simulink library "mylib"  (Simulink 9.2)
settings: Solver=VariableStepAuto  StartTime=0.0  StopTime=10.0  RelTol=1e-3
values from neighbouring files (symbols this model uses):
  FLINT32_MAX = flintmax('single')    [lib_consts.m]
undefined symbols (not defined in the file or in its folder): BAR_2_Pa, CC_2_M3, CCpREV_2_M3pRAD, DEG_2_RAD, DiscIntNeverNeededParam, G_2_MPS2, KNOTS_2_KPH, KPH_2_KNOTS, KPH_2_MPS, kXX_2_XX, M3_2_CC, M3pRAD_2_CCpREV, MPS2_2_G, MPS_2_KPH, Pa_2_BAR, RAD_2_DEG, RADpS_2_RPM, RPM_2_RADpS, XX_2_kXX
libraries: $bdroot x12, simulink x4, Ricardo_SW_dev_lib x1
(part 1 of 2)
settings Model: Creator=Gavin  LastModifiedBy=Gavin

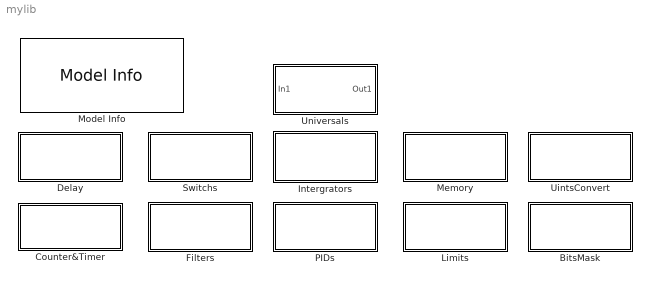
== system mylib ==
  BitsMask : Subsystem
      mask Display:
      | name = gcb;
      | str_id = strfind(gcb,'/');
      | name_mask = name(str_id+1:end);
      | disp([name_mask,'\nBlocks']);
      | color('black')
  Counter&Timer : Subsystem
      mask Display:
      | name = gcb;
      | str_id = strfind(gcb,'/');
      | name_mask = name(str_id+1:end);
      | disp([name_mask,'\nBlocks']);
      | color('black')
  Delay : Subsystem
      mask Display:
      | name = gcb;
      | str_id = strfind(gcb,'/');
      | name_mask = name(str_id+1:end);
      | disp([name_mask,'\nBlocks']);
      | color('black')
  Filters : Subsystem
      mask Display:
      | name = gcb;
      | str_id = strfind(gcb,'/');
      | name_mask = name(str_id+1:end);
      | disp([name_mask,'\nBlocks']);
      | color('black')
  Intergrators : Subsystem
      mask Display:
      | name = gcb;
      | str_id = strfind(gcb,'/');
      | name_mask = name(str_id+1:end);
      | disp([name_mask,'\nBlocks']);
      | color('black')
  Limits : Subsystem
      mask Display:
      | name = gcb;
      | str_id = strfind(gcb,'/');
      | name_mask = name(str_id+1:end);
      | disp([name_mask,'\nBlocks']);
      | color('black')
  Memory : Subsystem
      mask Display:
      | name = gcb;
      | str_id = strfind(gcb,'/');
      | name_mask = name(str_id+1:end);
      | disp([name_mask,'\nBlocks']);
      | color('black')
  Model Info : simulink/Model-Wide Utilities/Model Info  Frame=on  DisplayStringWithTags=|  HorizontalTextAlignment=Center  LeftAlignmentValue=0.5
      | Model:%<ModelName>
      | Create:%<Creator>
      | Time:%<Created>
      | ------------------------------------------------------
      | Modify:%<LastModifiedBy>
      | Time:%<LastModificationDate>
  PIDs : Subsystem
      mask Display:
      | name = gcb;
      | str_id = strfind(gcb,'/');
      | name_mask = name(str_id+1:end);
      | disp([name_mask,'\nBlocks']);
      | color('black')
  Switchs : Subsystem
      mask Display:
      | name = gcb;
      | str_id = strfind(gcb,'/');
      | name_mask = name(str_id+1:end);
      | disp([name_mask,'\nBlocks']);
      | color('black')
  UintsConvert : Subsystem
      mask Display:
      | name = gcb;
      | str_id = strfind(gcb,'/');
      | name_mask = name(str_id+1:end);
      | disp([name_mask,'\nBlocks']);
      | color('black')
  Universals : Subsystem
      mask Display:
      | name = gcb;
      | str_id = strfind(gcb,'/');
      | name_mask = name(str_id+1:end);
      | disp([name_mask,'\nBlocks']);
      | color('black')

== system mylib/BitsMask ==
  note: Bin2Dec
  bitmask16 : Subsystem
  bitmask32 : Subsystem
  bitmask8 : Subsystem

== system mylib/Counter&Timer ==
  Counter_Down : Subsystem
  Counter_Up : Subsystem
  RollingCounter : Subsystem
  Timer : Subsystem
  rolling_edge_counter : Subsystem

== system mylib/Delay ==
  debounce : Subsystem  TreatAsAtomicUnit=on
  turnOFF_delay : Subsystem  TreatAsAtomicUnit=on
  turnON_delay : Subsystem  TreatAsAtomicUnit=on

== system mylib/Filters ==
  1st Order Filter : Subsystem

== system mylib/Intergrators ==
  Accumulator : Subsystem  mask{InitValue=0}
      mask prompts: InitValue "Initial Value"
  Accumulator_Limit : Subsystem  mask{InitValue=0}
      mask prompts: InitValue "Initial Value"
  Intergrator_K : Subsystem  mask{InitValue=0, Parameter2=Inherit: auto}
      mask prompts: InitValue "Initial Value"
  Intergrator_T : Subsystem  mask{InitValue=0}
      mask prompts: InitValue "Initial Value"

== system mylib/Limits ==
  MaxMin_Limit : Subsystem
  RateLimit : Subsystem

== system mylib/Memory ==
  DoubleEdge_Detect : Subsystem
  Falling_Detect : Subsystem
  Rising_Detect : Subsystem
  SR_latch : Subsystem  TreatAsAtomicUnit=on  RTWFcnName=ff_resetting
      settings: RTWFcnNameOpts=Use subsystem name

== system mylib/PIDs ==
  PI_FeedForward : Subsystem  TreatAsAtomicUnit=on
      settings: RTWSystemCode=Nonreusable function
  PI_adjustable : Subsystem  TreatAsAtomicUnit=on
      settings: RTWSystemCode=Nonreusable function

== system mylib/Switchs ==
  Save_Value : Subsystem  mask{initvalue=0}
      mask prompts: initvalue "Inital Value"
  Selector : Subsystem
  switch_ramp : Subsystem  TreatAsAtomicUnit=on  RTWFcnName=SwitchRamp  mask(Switch Ramp){RampExecTimeCal=0.01}
      mask prompts: RampExecTimeCal "Execution Time"
      mask help:
      | Pass through input 1 when input 2 is different from 0; otherwise pass input 3.
      |
      | The first and third ports are data ports, and the second input port is the control port.
      | The criteria for control port 2 is u2 ~= 0.
      |
      | When the control port u2 changes state, the output doesn't switch immediately to the
      | selected data port, but a rate limiter is applied.
      |
      | Limit rising and falling rates of the signal by using the fourth input (upper limit)
      | and fifth input (lower limit).
      mask init:
      | RampExecTime = max(RampExecTimeCal, 0.001);
      settings: AttributesFormatString=%<RampExecTimeCal>  RTWFcnNameOpts=Use subsystem name  RTWFileNameOpts=Use subsystem name
      mask Display:
      | x1 = [.1 .4]; y1 = [.9 .9];
      | x2 = [.1 .4]; y2 = [.5 .5];
      | x3 = [.4 .4 .44 .44 .4]; y3 = [.87 .93 .93 .87 .87];
      | x4 = [.4 .4 .44 .44 .4]; y4 = [.47 .53 .53 .47 .47];
      | x5 = [.1 .2]; y5 = [.7 .7];
      | x6 = [.2 .2]; y6 = [.65 .75];
      | text(.25, .7, '~=0');
      | x7 = [.42 .7 .9]; y7 = [.9 .7 .7];
      | 
      | x8 = [.2 .8]; y8 = [.2 .2];
      | x9 = [.5 .5]; y9 = [0 .4];
      | x10 = [.25 .75]; y10 = [0.05 .35];
      | 
      | plot(x1,y1,x2,y2,x3,y3,x4,y4,x5,y5,x6,y6,x7,y7,x8,y8,x9,y9,x10,y10);

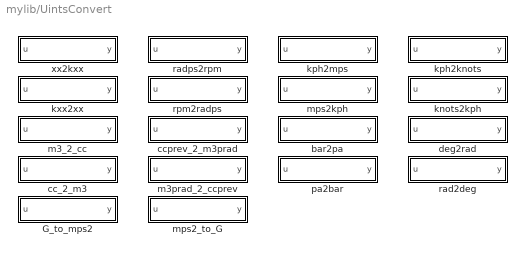
== system mylib/UintsConvert ==
  G_to_mps2 : Subsystem  mask(Conversion){}
      mask help: Convert acceleration in G to Meters per Second squared
      mask Display: disp('G \rightarrow m/s^2', 'texmode', 'on')
  bar2pa : Subsystem  mask(Conversion){}
      mask help: Converts bar to Pascals
      mask Display: disp('bar \rightarrow Pa', 'texmode', 'on')
  cc_2_m3 : Subsystem  mask(Conversion){}
      mask help: Converts cubic centimetres to cubic metres
      mask Display: disp('cc \rightarrow m3', 'texmode', 'on')
  ccprev_2_m3prad : Subsystem  mask(Conversion){}
      mask help: Converts cubic centimetres per revolution to metres cubed per radian
      mask Display: disp('cc/rev \rightarrow m3/rad', 'texmode', 'on')
  deg2rad : Subsystem
      mask help: Converts degrees to radians
      mask Display: disp('deg \rightarrow rad', 'texmode', 'on')
  knots2kph : Subsystem  mask(Conversion){}
      mask help: Convert knots to kilometres per hour
      mask Display: disp('knots \rightarrow kph', 'texmode', 'on')
  kph2knots : Subsystem  mask(Conversion){}
      mask help: Convert kilometres per hour to knots
      mask Display: disp('kph \rightarrow knots', 'texmode', 'on')
  kph2mps : Subsystem  mask(Conversion){}
      mask help: Convert Kilometers per hour to Meters per second
      mask Display: disp('kph \rightarrow m/s', 'texmode', 'on')
  kxx2xx : Subsystem  mask(Conversion){}
      mask help: Multiply by 1000.
      mask Display: disp('kiloxx \rightarrow xx', 'texmode', 'on')
  m3_2_cc : Subsystem  mask(Conversion){}
      mask help: Converts cubic metres to cubic centimetres
      mask Display: disp('m3 \rightarrow cc', 'texmode', 'on')
  m3prad_2_ccprev : Subsystem  mask(Conversion){}
      mask help: Converts metres cubed per radian to cubic centimetres per rev
      mask Display: disp('m3/rad \rightarrow cc/rev', 'texmode', 'on')
  mps2_to_G : Subsystem  mask(Conversion){}
      mask help: Convert acceleration in Meters per Second squared to G
      mask Display: disp('m/s^2 \rightarrow G', 'texmode', 'on')
  mps2kph : Subsystem  mask(Conversion){}
      mask help: Convert metres per second to kilometres per hour
      mask Display: disp('m/s \rightarrow kph', 'texmode', 'on')
  pa2bar : Subsystem  mask(Conversion){}
      mask help: Converts Pascals to bar
      mask Display: disp('Pa \rightarrow bar', 'texmode', 'on')
  rad2deg : Subsystem
      mask help: Converts radians to degrees
      mask Display: disp('rad \rightarrow deg', 'texmode', 'on')
  radps2rpm : Subsystem
      mask help: Converts radians per second to revolutions per minute.
      mask Display: disp('rad/s \rightarrow rpm', 'texmode', 'on')
  rpm2radps : Subsystem
      mask help: Converts revolutions per minute to radians per second.
      mask Display: disp('rpm \rightarrow rad/s', 'texmode', 'on')
  xx2kxx : Subsystem  mask(Conversion){}
      mask help: Divides by 1000.
      mask Display: disp('xx \rightarrow kiloxx', 'texmode', 'on')

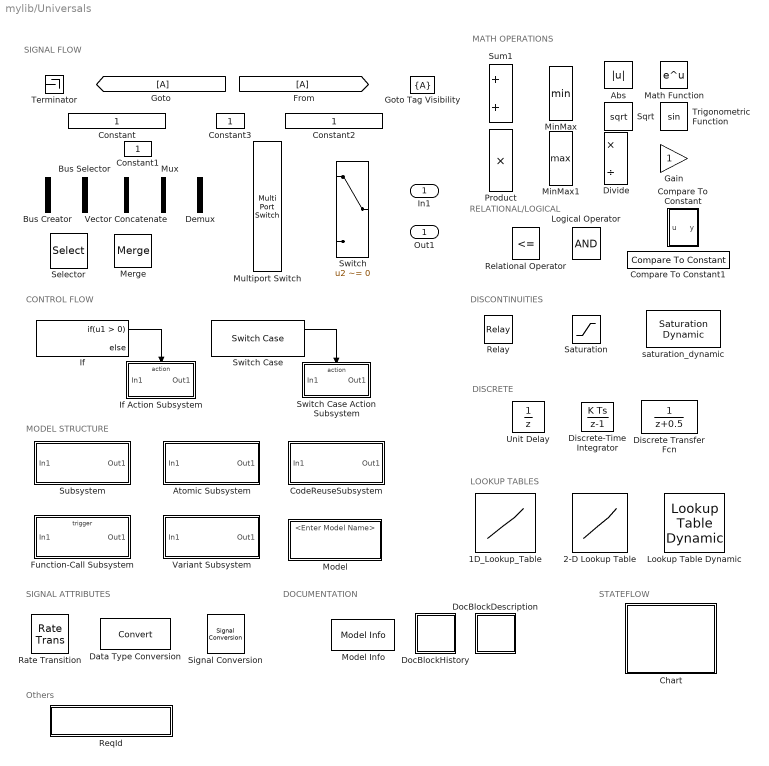
== system mylib/Universals ==
  note: Others
  note: STATEFLOW
  note: DOCUMENTATION
  note: SIGNAL ATTRIBUTES
  note: LOOKUP TABLES
  note: DISCRETE
  note: DISCONTINUITIES
  note: RELATIONAL/LOGICAL
  note: MATH OPERATIONS
  note: MODEL STRUCTURE
  note: CONTROL FLOW
  note: SIGNAL FLOW
  In1 : Inport
  1D_Lookup_Table : Lookup_n-D  NumberOfTableDimensions=1  BreakpointsForDimension1=[-5:5]  Table=tanh([-5:5])  ExtrapMethod=Clip  UseLastTableValue=on  InternalRulePriority=Speed  RndMeth=Zero  InputSameDT=on
      settings: AttributesFormatString=<input=%<BreakpointsForDimension1>>\n<output=%<Table>>
  2-D Lookup Table : Lookup_n-D  BreakpointsForDimension1=[1:3]  BreakpointsForDimension2=[1:3]  TableDataTypeStr=Inherit: Inherit from 'Table data'  ExtrapMethod=Clip  UseLastTableValue=on  InternalRulePriority=Speed  OutDataTypeStr=Inherit: Inherit from 'Table data'  RndMeth=Zero
      settings: AttributesFormatString=|
      | <row=%<BreakpointsForDimension1>>
      | <column=%<BreakpointsForDimension2>>
      | <table=%<Table>>
  Abs : Abs  OutDataTypeStr=single  RndMeth=Zero
  Atomic Subsystem : Subsystem  TreatAsAtomicUnit=on
  Bus Creator : BusCreator  Inputs=2
  Bus Selector : BusSelector  OutputSignals=signal1,signal2
  Chart : Stateflow chart  TreatAsAtomicUnit=on
  CodeReuseSubsystem : Subsystem  TreatAsAtomicUnit=on
      settings: RTWFcnNameOpts=Use subsystem name  RTWFileNameOpts=Use function name
  Compare To Constant : Subsystem  mask(Compare To Constant){relop===, const=3}
      mask prompts: relop "Operator:"; const "Constant value:"
      mask help: Determine how a signal compares to a constant.
      mask init:
      | blkName = gcb;
      | 
      | set_param([blkName,'/Compare'],'relop',relop);
      | 
      | const_str = get_param(blkName, 'const');
      | 
      | str = [relop, ' ', const_str];
      mask TypeOptions relop: == | ~= | < | <= | >= | >
      mask Display: disp(str)
  Compare To Constant1 : $bdroot/Universals/Compare To Constant  relop===  const=3
  Constant{,1..3} (4 alike) : Constant  SampleTime=-1
      Constant settings: AttributesFormatString=<%<OutDataTypeStr>>
      Constant1 settings: AttributesFormatString=<%<OutDataTypeStr>>
  Data Type Conversion : DataTypeConversion  RndMeth=Zero
  Demux : Demux  Outputs=2
  Discrete Transfer Fcn : DiscreteTransferFcn  SampleTime=1  RndMeth=Zero
      settings: AttributesFormatString=<tsample=%<sampleTime>>
  Discrete-Time Integrator : DiscreteIntegrator  RndMeth=Zero  ICPrevOutput=DiscIntNeverNeededParam  ICPrevScaledInput=DiscIntNeverNeededParam
      settings: AttributesFormatString=<initial=%<initialcondition>>\n<tsample=%<sampleTime>>\n<limits=%<UpperSaturationLimit>/%<LowerSaturationLimit>(%<LimitOutput>)>
  Divide : Product  Inputs=*/
  DocBlockDescription : Subsystem  mask(DocBlock){ECoderFlag=Description, DocumentType=Text}
      mask prompts: ECoderFlag "RTW Embedded Coder Flag"; DocumentType "Document Type"
      mask help: Use this block to save long descriptive text with the model. Double-clicking the block will open an editor.
      settings: AttributesFormatString=%<ECoderFlag>  DeleteFcn=docblock('close_document',gcb);  PreSaveFcn=docblock('save_document',gcb);  OpenFcn=docblock('edit_document',gcb);
      mask TypeOptions DocumentType: Text | RTF | HTML
      mask Display:
      | plot([.8 0 0 1 1 .8 .8 1],[1 1 0 0 .8 1 .8 .8]);
      | text(.5,.6,'DOC','horizontalalignment','center');
      | text(.95,.05,get_param(gcb,'DocumentType'),'verticalalignment','bottom','horizontalalignment','right');
  DocBlockHistory : Subsystem  mask(DocBlock){ECoderFlag=History, DocumentType=Text}
      mask prompts: ECoderFlag "RTW Embedded Coder Flag"; DocumentType "Document Type"
      mask help: Use this block to save long descriptive text with the model. Double-clicking the block will open an editor.
      settings: AttributesFormatString=%<ECoderFlag>  DeleteFcn=docblock('close_document',gcb);  PreSaveFcn=docblock('save_document',gcb);  OpenFcn=docblock('edit_document',gcb);
      mask TypeOptions DocumentType: Text | RTF | HTML
      mask Display:
      | plot([.8 0 0 1 1 .8 .8 1],[1 1 0 0 .8 1 .8 .8]);
      | text(.5,.6,'DOC','horizontalalignment','center');
      | text(.95,.05,get_param(gcb,'DocumentType'),'verticalalignment','bottom','horizontalalignment','right');
  Function-Call Subsystem : Subsystem  TreatAsAtomicUnit=on
  Gain : Gain  RndMeth=Zero
  Goto Tag Visibility : GotoTagVisibility
  If : If
  If Action Subsystem : Subsystem  TreatAsAtomicUnit=on
  Logical Operator : Logic  AllPortsSameDT=off  OutDataTypeStr=boolean
  Lookup Table Dynamic : simulink/Lookup Tables/Lookup Table Dynamic  LookUpMeth=Interpolation-Use End Values  OutDataType=fixdt('single')  OutScaling=[]  OutputDataTypeScalingMode=Specify via dialog  OutDataTypeStr=fixdt('single')  RndMeth=Zero  DoSatur=off
      settings: SourceProductName=Simulink
  Math Function : Math  SaturateOnIntegerOverflow=on
  Merge : Merge
      settings: AttributesFormatString=<initial=%<initialoutput>>
  MinMax : MinMax  Inputs=2  OutDataTypeStr=single  RndMeth=Zero
  MinMax1 : MinMax  Function=max  Inputs=2  OutDataTypeStr=single  RndMeth=Zero
  Model : ModelReference
  Model Info : simulink/Model-Wide Utilities/Model Info  Frame=on  DisplayStringWithTags=Model Info  HorizontalTextAlignment=Center  LeftAlignmentValue=0.5
  Multiport Switch : MultiPortSwitch  DiagnosticForDefault=Warning  RndMeth=Zero  InputSameDT=on
  Mux : Mux  Inputs=2
  Product : Product  RndMeth=Zero
  Rate Transition : RateTransition
  Relational Operator : RelationalOperator  Operator=<=  OutDataTypeStr=boolean  RndMeth=Nearest
  Relay : Relay  ZeroCross=off
      settings: AttributesFormatString=<high=(%<onswitchvalue>,%<onoutputvalue>)>\n<low=(%<offswitchvalue>,%<offoutputvalue>)>
  ReqId : Subsystem  mask(ReqId){req_str=SRS_555}
      mask prompts: req_str "Requirement:"
      mask help: Requirement Id
      mask Display: disp(sprintf('ReqId: %s',req_str));
  Saturation : Saturate  RndMeth=Zero
      settings: AttributesFormatString=<limits=%<upperlimit>\%<lowerlimit>>
  Selector : Selector  InputPortWidth=3  IndexOptions=Index vector (dialog)  Indices=[1 3]  OutputSizes=1
  Signal Conversion : SignalConversion  OverrideOpt=off
  Sqrt : Sqrt  RndMeth=Zero
  Subsystem : Subsystem
  Sum1 : Sum  RndMeth=Zero
  Switch : Switch  Criteria=u2 ~= 0  Threshold=0.5  RndMeth=Zero
      settings: AttributesFormatString=<threshold=%<threshold>>\n<criteria=%<Criteria>>
  Switch Case : SwitchCase
  Switch Case Action Subsystem : Subsystem  TreatAsAtomicUnit=on
  Terminator : Terminator
  Trigonometric Function : Trigonometry
  Unit Delay : UnitDelay  SampleTime=-1
      settings: AttributesFormatString=<initial=%<x0>>
  Variant Subsystem : Subsystem  Variant=on
  Vector Concatenate : Concatenate
  saturation_dynamic : simulink/Discontinuities/Saturation Dynamic  OutMin=[]  OutMax=[]  OutDataTypeStr=Inherit: Same as second input  OutDataType=fixdt(1, 16)  OutScaling=2^-10  RndMeth=Zero  DoSatur=off
  Out1 : Outport
  wires:
  Switch Case/1 -> Switch Case Action Subsystem/Action
  If/1 -> If Action Subsystem/Action

== system mylib/BitsMask/bitmask16 ==
  note: Take a vector of booleans and turn it into a single integer mask
  data : Inport
      settings: AttributesFormatString=<tsample=%<SampleTime>>
  Constant : Constant  Value=uint8(16)  SampleTime=-1
      settings: AttributesFormatString=<tsample=%<SampleTime>>
  Data Type Conversion : DataTypeConversion  OutDataTypeStr=uint16  RndMeth=Zero
  MinMax : MinMax  Inputs=2
  Signal Specification : SignalSpecification  OutDataTypeStr=boolean
  Width : Width  DataType=uint8
  mask16 : Stateflow chart  TreatAsAtomicUnit=on
  result : Outport
      settings: AttributesFormatString=<tsample=%<SampleTime>>
  wires:
  data/1 -> Width/1, Signal Specification/1
  MinMax/1 -> mask16/2(num_bits)
  Constant/1 -> MinMax/2
  mask16/1(result) -> result/1
  Width/1 -> MinMax/1
  Data Type Conversion/1 -> mask16/1(data)
  Signal Specification/1 -> Data Type Conversion/1

== system mylib/BitsMask/bitmask32 ==
  note: Take a vector of booleans and turn it into a single integer mask
  data : Inport
      settings: AttributesFormatString=<tsample=%<SampleTime>>
  Constant : Constant  Value=uint8(32)  SampleTime=-1
      settings: AttributesFormatString=<tsample=%<SampleTime>>
  Data Type Conversion : DataTypeConversion  OutDataTypeStr=uint32  RndMeth=Zero
  MinMax : MinMax  Inputs=2
  Signal Specification : SignalSpecification  OutDataTypeStr=boolean
  Width : Width  DataType=uint8
  mask32 : Stateflow chart  TreatAsAtomicUnit=on
  result : Outport
      settings: AttributesFormatString=<tsample=%<SampleTime>>
  wires:
  data/1 -> Width/1, Signal Specification/1
  MinMax/1 -> mask32/2(num_bits)
  Constant/1 -> MinMax/2
  mask32/1(result) -> result/1
  Width/1 -> MinMax/1
  Data Type Conversion/1 -> mask32/1(data)
  Signal Specification/1 -> Data Type Conversion/1

== system mylib/BitsMask/bitmask8 ==
  note: Take a vector of booleans and turn it into a single integer mask
  data : Inport
      settings: AttributesFormatString=<tsample=%<SampleTime>>
  Constant : Constant  Value=uint8(8)  SampleTime=-1
      settings: AttributesFormatString=<tsample=%<SampleTime>>
  Data Type Conversion : DataTypeConversion  OutDataTypeStr=uint8  RndMeth=Zero
  MinMax : MinMax  Inputs=2
  Signal Specification : SignalSpecification  OutDataTypeStr=boolean
  Width : Width  DataType=uint8
  mask8 : Stateflow chart  TreatAsAtomicUnit=on
  result : Outport
      settings: AttributesFormatString=<tsample=%<SampleTime>>
  wires:
  Signal Specification/1 -> Data Type Conversion/1
  Data Type Conversion/1 -> mask8/1(data)
  Width/1 -> MinMax/1
  mask8/1(result) -> result/1
  Constant/1 -> MinMax/2
  MinMax/1 -> mask8/2(num_bits)
  data/1 -> Signal Specification/1, Width/1

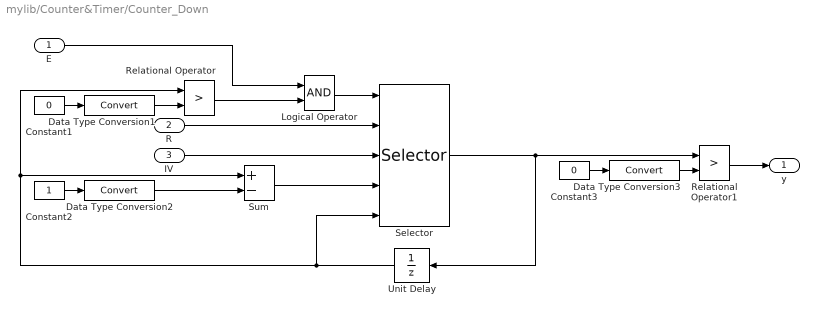
== system mylib/Counter&Timer/Counter_Down ==
  E : Inport
  R : Inport  Port=2
  IV : Inport  Port=3
  Constant1 : Constant  Value=0
  Constant2 : Constant
  Constant3 : Constant  Value=0
  Data Type Conversion1 : DataTypeConversion
  Data Type Conversion2 : DataTypeConversion
  Data Type Conversion3 : DataTypeConversion
  Logical Operator : Logic  AllPortsSameDT=off  OutDataTypeStr=boolean
  Relational Operator : RelationalOperator  Operator=>  OutDataTypeStr=boolean  RndMeth=Nearest
  Relational Operator1 : RelationalOperator  Operator=>  OutDataTypeStr=boolean  RndMeth=Nearest
  Selector : $bdroot/Switchs/Selector  SystemSampleTime=-1
  Sum : Sum  Inputs=+-  RndMeth=Zero
  Unit Delay : UnitDelay  InitialCondition=1  SampleTime=-1
      settings: AttributesFormatString=<initial=%<x0>>\n<tsample=%<sampleTime>>
  y : Outport
  wires:
  Unit Delay/1 -> Sum/1, Relational Operator/1, Selector/5
  Sum/1 -> Selector/4
  E/1 -> Logical Operator/1
  Selector/1 -> Relational Operator1/1, Unit Delay/1
  R/1 -> Selector/2
  Logical Operator/1 -> Selector/1
  Relational Operator/1 -> Logical Operator/2
  Constant1/1 -> Data Type Conversion1/1
  Data Type Conversion1/1 -> Relational Operator/2
  Constant2/1 -> Data Type Conversion2/1
  Data Type Conversion2/1 -> Sum/2
  IV/1 -> Selector/3
  Relational Operator1/1 -> y/1
  Constant3/1 -> Data Type Conversion3/1
  Data Type Conversion3/1 -> Relational Operator1/2

== system mylib/Counter&Timer/Counter_Up ==
  E : Inport
  R : Inport  Port=2
  IV : Inport  Port=3
  Constant2 : Constant
  Constant3 : Constant  Value=0
  Data Type Conversion2 : DataTypeConversion
  Data Type Conversion3 : DataTypeConversion
  Delay_IV : Subsystem
  Relational Operator1 : RelationalOperator  Operator=>  OutDataTypeStr=boolean  RndMeth=Nearest
  Selector : $bdroot/Switchs/Selector  SystemSampleTime=-1
  Sum : Sum  Inputs=+-  RndMeth=Zero
  y : Outport
  wires:
  Data Type Conversion3/1 -> Relational Operator1/2
  Constant3/1 -> Data Type Conversion3/1
  Relational Operator1/1 -> y/1
  IV/1 -> Delay_IV/2(IV), Selector/3
  Data Type Conversion2/1 -> Sum/2
  Constant2/1 -> Data Type Conversion2/1
  E/1 -> Selector/1
  R/1 -> Selector/2
  Selector/1 -> Delay_IV/1(u), Relational Operator1/1
  Sum/1 -> Selector/4
  Delay_IV/1(y) -> Selector/5, Sum/1

== system mylib/Counter&Timer/RollingCounter ==
  Add : Sum  Inputs=++|
  Constant : Constant  OutDataTypeStr=uint8
  Constant1 : Constant  Value=14  OutDataTypeStr=uint8
  Constant2 : Constant  Value=0  OutDataTypeStr=uint8
  Relational Operator : RelationalOperator  Operator=<=  OutDataTypeStr=boolean  RndMeth=Nearest
  Switch : Switch  Criteria=u2 > Threshold  OutDataTypeStr=uint8
  Unit Delay : UnitDelay  SampleTime=-1
  out : Outport
  wires:
  Constant/1 -> Add/2
  Constant1/1 -> Relational Operator/2
  Add/1 -> Switch/1
  Relational Operator/1 -> Switch/2
  Constant2/1 -> Switch/3
  Unit Delay/1 -> out/1, Relational Operator/1, Add/1
  Switch/1 -> Unit Delay/1

== system mylib/Counter&Timer/Timer ==
  E : Inport
  R : Inport  Port=2
  dT : Inport  Port=3
  Constant : Constant  Value=0
  Data Type Conversion : DataTypeConversion
  Selector : $bdroot/Switchs/Selector  SystemSampleTime=-1
  Sum : Sum  RndMeth=Zero
  Unit Delay : UnitDelay  SampleTime=-1
      settings: AttributesFormatString=<initial=%<x0>>\n<tsample=%<sampleTime>>
  timer_out : Outport
  wires:
  R/1 -> Selector/2
  Selector/1 -> Unit Delay/1, timer_out/1
  Constant/1 -> Data Type Conversion/1
  Data Type Conversion/1 -> Selector/3
  E/1 -> Selector/1
  Sum/1 -> Selector/4
  dT/1 -> Sum/1
  Unit Delay/1 -> Selector/5, Sum/2

== system mylib/Counter&Timer/rolling_edge_counter ==
  note: Increment a rolling counter each time a false -> true transition is detected on the input
  input_flg : Inport  OutDataTypeStr=boolean
      settings: AttributesFormatString=|
      | <tsample=%<SampleTime>>
      | <DataType=%<OutDataTypeStr>>
  boolean_edge : Subsystem
  conditional_counter : Subsystem
  rolling_ctr : Outport
      settings: AttributesFormatString=<tsample=%<SampleTime>>
  wires:
  input_flg/1 -> boolean_edge/1(input_flg)  "input_flg"
  conditional_counter/1(rolling_ctr) -> rolling_ctr/1
  boolean_edge/1(edgle_flg) -> conditional_counter/1(increment_on)

== system mylib/Delay/debounce ==
  flg_in : Inport
      settings: AttributesFormatString=<tsample=%<SampleTime>>
  t_delay_on : Inport  Port=2
      settings: AttributesFormatString=<tsample=%<SampleTime>>
  t_delay_off : Inport  Port=3
      settings: AttributesFormatString=<tsample=%<SampleTime>>
  t_step : Inport  Port=4
      settings: AttributesFormatString=<tsample=%<SampleTime>>
  Data Type Conversion : DataTypeConversion  OutDataTypeStr=boolean
  Saturation : Saturate  UpperLimit=FLINT32_MAX  LowerLimit=0  RndMeth=Zero
      settings: AttributesFormatString=<limits=%<upperlimit>\%<lowerlimit>>
  Saturation1 : Saturate  UpperLimit=FLINT32_MAX  LowerLimit=0  RndMeth=Zero
      settings: AttributesFormatString=<limits=%<upperlimit>\%<lowerlimit>>
  timed_debounce : Stateflow chart  TreatAsAtomicUnit=on
  flg_out : Outport
      settings: AttributesFormatString=<tsample=%<SampleTime>>
  wires:
  Data Type Conversion/1 -> timed_debounce/1(flg_in)
  t_delay_off/1 -> Saturation1/1
  Saturation1/1 -> timed_debounce/3(t_delay_off)  "t_delay_off"
  t_delay_on/1 -> Saturation/1
  flg_in/1 -> Data Type Conversion/1
  t_step/1 -> timed_debounce/4(t_step)
  timed_debounce/1(flg_out) -> flg_out/1
  Saturation/1 -> timed_debounce/2(t_delay_on)  "t_delay_on"

== system mylib/Delay/turnOFF_delay ==
  flg_in : Inport
      settings: AttributesFormatString=<tsample=%<SampleTime>>
  t_delay_off : Inport  Port=2
      settings: AttributesFormatString=<tsample=%<SampleTime>>
  t_step : Inport  Port=3
      settings: AttributesFormatString=<tsample=%<SampleTime>>
  Data Type Conversion : DataTypeConversion  OutDataTypeStr=boolean
  Saturation1 : Saturate  UpperLimit=FLINT32_MAX  LowerLimit=0  RndMeth=Zero
      settings: AttributesFormatString=<limits=%<upperlimit>\%<lowerlimit>>
  timed_delay : Stateflow chart  TreatAsAtomicUnit=on
  flg_out : Outport
      settings: AttributesFormatString=<tsample=%<SampleTime>>
  wires:
  timed_delay/1(flg_out) -> flg_out/1  "flg_out"
  t_step/1 -> timed_delay/3(t_step)  "t_step"
  flg_in/1 -> Data Type Conversion/1  "flg_in"
  Saturation1/1 -> timed_delay/2(t_delay_off)  "t_delay_off"
  t_delay_off/1 -> Saturation1/1  "t_delay_off"
  Data Type Conversion/1 -> timed_delay/1(flg_in)

== system mylib/Delay/turnON_delay ==
  flg_in : Inport
      settings: AttributesFormatString=<tsample=%<SampleTime>>
  t_delay_on : Inport  Port=2
      settings: AttributesFormatString=<tsample=%<SampleTime>>
  t_step : Inport  Port=3
      settings: AttributesFormatString=<tsample=%<SampleTime>>
  Data Type Conversion : DataTypeConversion  OutDataTypeStr=boolean
  Saturation : Saturate  UpperLimit=FLINT32_MAX  LowerLimit=0  RndMeth=Zero
      settings: AttributesFormatString=<limits=%<upperlimit>\%<lowerlimit>>
  timed_delay : Stateflow chart  TreatAsAtomicUnit=on
  flg_out : Outport
      settings: AttributesFormatString=<tsample=%<SampleTime>>
  wires:
  Saturation/1 -> timed_delay/2(t_delay_on)  "t_delay_on"
  timed_delay/1(flg_out) -> flg_out/1  "flg_out"
  t_step/1 -> timed_delay/3(t_step)  "t_step"
  flg_in/1 -> Data Type Conversion/1  "flg_in"
  t_delay_on/1 -> Saturation/1  "t_delay_on"
  Data Type Conversion/1 -> timed_delay/1(flg_in)

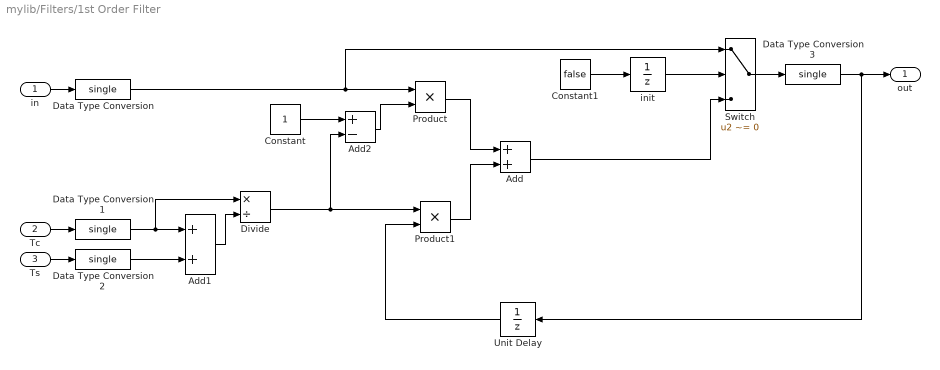
== system mylib/Filters/1st Order Filter ==
  in : Inport
  Tc : Inport  Port=2
  Ts : Inport  Port=3
  Add : Sum
  Add1 : Sum
  Add2 : Sum  Inputs=+-
  Constant : Constant  OutDataTypeStr=single
  Constant1 : Constant  Value=false
  Data Type Conversion{,1..3} (4 alike) : DataTypeConversion  OutDataTypeStr=single
  Divide : Product  Inputs=*/
  Product : Product  RndMeth=Zero
  Product1 : Product  RndMeth=Zero
  Switch : Switch  Criteria=u2 ~= 0
  Unit Delay : UnitDelay  SampleTime=-1
  init : UnitDelay  InitialCondition=true  SampleTime=-1
      settings: AttributesFormatString=<X0=%<X0>>
  out : Outport
  wires:
  Unit Delay/1 -> Product1/2
  Tc/1 -> Data Type Conversion1/1
  Ts/1 -> Data Type Conversion2/1
  Add1/1 -> Divide/2
  Constant/1 -> Add2/1
  Divide/1 -> Add2/2, Product1/1
  in/1 -> Data Type Conversion/1
  Add2/1 -> Product/2
  Product/1 -> Add/1
  Product1/1 -> Add/2
  Constant1/1 -> init/1
  init/1 -> Switch/2
  Switch/1 -> Data Type Conversion3/1
  Add/1 -> Switch/3
  Data Type Conversion/1 -> Product/1, Switch/1
  Data Type Conversion1/1 -> Add1/1, Divide/1
  Data Type Conversion2/1 -> Add1/2
  Data Type Conversion3/1 -> out/1, Unit Delay/1

== system mylib/Intergrators/Accumulator ==
  u : Inport
  E : Inport  Port=2
  R : Inport  Port=3
  RV : Inport  Port=4
  dT : Inport  Port=5
  Product : Product  RndMeth=Zero
  Selector : $bdroot/Switchs/Selector  SystemSampleTime=-1
  Sum : Sum  RndMeth=Zero
  Unit Delay : UnitDelay  InitialCondition=InitValue  SampleTime=-1
      settings: AttributesFormatString=<initial=%<x0>>\n<tsample=%<sampleTime>>
  out : Outport
  wires:
  E/1 -> Selector/1
  R/1 -> Selector/2
  RV/1 -> Selector/3
  u/1 -> Product/1
  Sum/1 -> Selector/4
  Unit Delay/1 -> Selector/5, Sum/2
  Selector/1 -> Unit Delay/1, out/1
  Product/1 -> Sum/1
  dT/1 -> Product/2

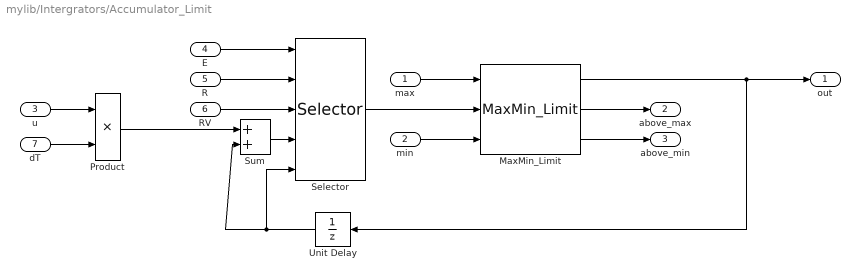
== system mylib/Intergrators/Accumulator_Limit ==
  max : Inport
  min : Inport  Port=2
  u : Inport  Port=3
  E : Inport  Port=4
  R : Inport  Port=5
  RV : Inport  Port=6
  dT : Inport  Port=7
  MaxMin_Limit : $bdroot/Limits/MaxMin_Limit  SystemSampleTime=-1
  Product : Product  RndMeth=Zero
  Selector : $bdroot/Switchs/Selector  SystemSampleTime=-1
  Sum : Sum  RndMeth=Zero
  Unit Delay : UnitDelay  InitialCondition=InitValue  SampleTime=-1
      settings: AttributesFormatString=<initial=%<x0>>\n<tsample=%<sampleTime>>
  out : Outport
  above_max : Outport  Port=2
  above_min : Outport  Port=3
  wires:
  MaxMin_Limit/3 -> above_min/1
  MaxMin_Limit/1 -> Unit Delay/1, out/1
  Selector/1 -> MaxMin_Limit/2
  MaxMin_Limit/2 -> above_max/1
  min/1 -> MaxMin_Limit/3
  max/1 -> MaxMin_Limit/1
  E/1 -> Selector/1
  R/1 -> Selector/2
  RV/1 -> Selector/3
  u/1 -> Product/1
  Sum/1 -> Selector/4
  Unit Delay/1 -> Selector/5, Sum/2
  dT/1 -> Product/2
  Product/1 -> Sum/1

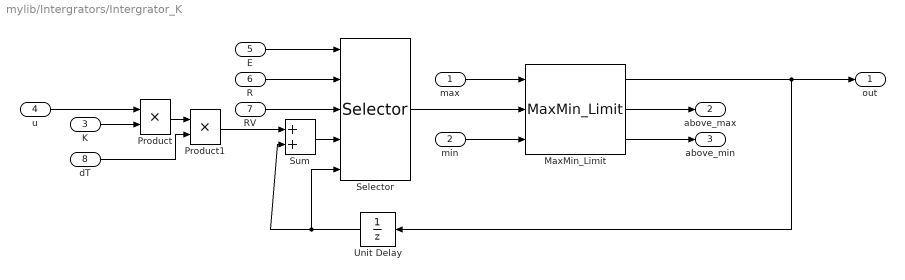
== system mylib/Intergrators/Intergrator_K ==
  max : Inport
  min : Inport  Port=2
  K : Inport  Port=3
  u : Inport  Port=4
  E : Inport  Port=5
  R : Inport  Port=6
  RV : Inport  Port=7
  dT : Inport  Port=8
  MaxMin_Limit : $bdroot/Limits/MaxMin_Limit  SystemSampleTime=-1
  Product : Product  RndMeth=Zero
  Product1 : Product  RndMeth=Zero
  Selector : $bdroot/Switchs/Selector  SystemSampleTime=-1
  Sum : Sum  RndMeth=Zero
  Unit Delay : UnitDelay  InitialCondition=InitValue  SampleTime=-1
      settings: AttributesFormatString=<initial=%<x0>>\n<tsample=%<sampleTime>>
  out : Outport
  above_max : Outport  Port=2
  above_min : Outport  Port=3
  wires:
  Unit Delay/1 -> Sum/2, Selector/5
  Sum/1 -> Selector/4
  RV/1 -> Selector/3
  R/1 -> Selector/2
  E/1 -> Selector/1
  max/1 -> MaxMin_Limit/1
  min/1 -> MaxMin_Limit/3
  MaxMin_Limit/2 -> above_max/1
  Selector/1 -> MaxMin_Limit/2
  MaxMin_Limit/1 -> out/1, Unit Delay/1
  MaxMin_Limit/3 -> above_min/1
  u/1 -> Product/1
  K/1 -> Product/2
  Product1/1 -> Sum/1
  Product/1 -> Product1/1
  dT/1 -> Product1/2

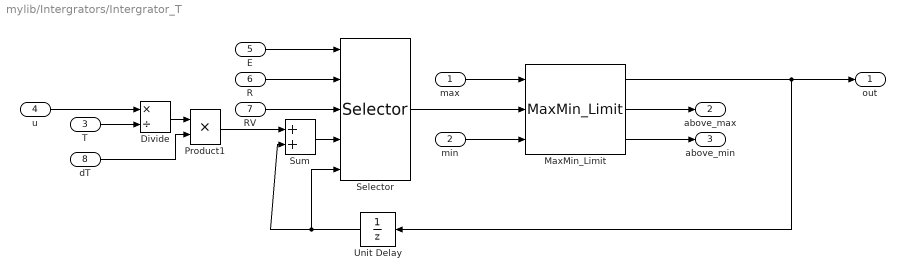
== system mylib/Intergrators/Intergrator_T ==
  max : Inport
  min : Inport  Port=2
  T : Inport  Port=3
  u : Inport  Port=4
  E : Inport  Port=5
  R : Inport  Port=6
  RV : Inport  Port=7
  dT : Inport  Port=8
  Divide : Product  Inputs=*/
  MaxMin_Limit : $bdroot/Limits/MaxMin_Limit  SystemSampleTime=-1
  Product1 : Product  RndMeth=Zero
  Selector : $bdroot/Switchs/Selector  SystemSampleTime=-1
  Sum : Sum  RndMeth=Zero
  Unit Delay : UnitDelay  InitialCondition=InitValue  SampleTime=-1
      settings: AttributesFormatString=<initial=%<x0>>\n<tsample=%<sampleTime>>
  out : Outport
  above_max : Outport  Port=2
  above_min : Outport  Port=3
  wires:
  dT/1 -> Product1/2
  Divide/1 -> Product1/1
  Product1/1 -> Sum/1
  T/1 -> Divide/2
  u/1 -> Divide/1
  MaxMin_Limit/3 -> above_min/1
  MaxMin_Limit/1 -> Unit Delay/1, out/1
  Selector/1 -> MaxMin_Limit/2
  MaxMin_Limit/2 -> above_max/1
  min/1 -> MaxMin_Limit/3
  max/1 -> MaxMin_Limit/1
  E/1 -> Selector/1
  R/1 -> Selector/2
  RV/1 -> Selector/3
  Sum/1 -> Selector/4
  Unit Delay/1 -> Selector/5, Sum/2

== system mylib/Limits/MaxMin_Limit ==
  max : Inport
      settings: AttributesFormatString=<tsample=%<SampleTime>>
  value : Inport  Port=2
      settings: AttributesFormatString=<tsample=%<SampleTime>>
  min : Inport  Port=3
      settings: AttributesFormatString=<tsample=%<SampleTime>>
  AboveMax : RelationalOperator  Operator=<  OutDataTypeStr=boolean  RndMeth=Nearest
  BelowMin : RelationalOperator  Operator=<  OutDataTypeStr=boolean  RndMeth=Nearest
  Switch : Switch  Criteria=u2 ~= 0  Threshold=0.5  RndMeth=Zero
      settings: AttributesFormatString=<threshold=%<threshold>>\n<criteria=%<Criteria>>
  Switch1 : Switch  Criteria=u2 ~= 0  Threshold=0.5  RndMeth=Zero
      settings: AttributesFormatString=<threshold=%<threshold>>\n<criteria=%<Criteria>>
  output : Outport
      settings: AttributesFormatString=<tsample=%<SampleTime>>
  above_max : Outport  Port=2
      settings: AttributesFormatString=<tsample=%<SampleTime>>
  below_min : Outport  Port=3
      settings: AttributesFormatString=<tsample=%<SampleTime>>
  wires:
  max/1 -> Switch/1, AboveMax/1
  value/1 -> AboveMax/2, Switch1/3, BelowMin/1
  AboveMax/1 -> Switch/2, above_max/1
  Switch/1 -> output/1
  min/1 -> Switch1/1, BelowMin/2
  Switch1/1 -> Switch/3
  BelowMin/1 -> below_min/1, Switch1/2

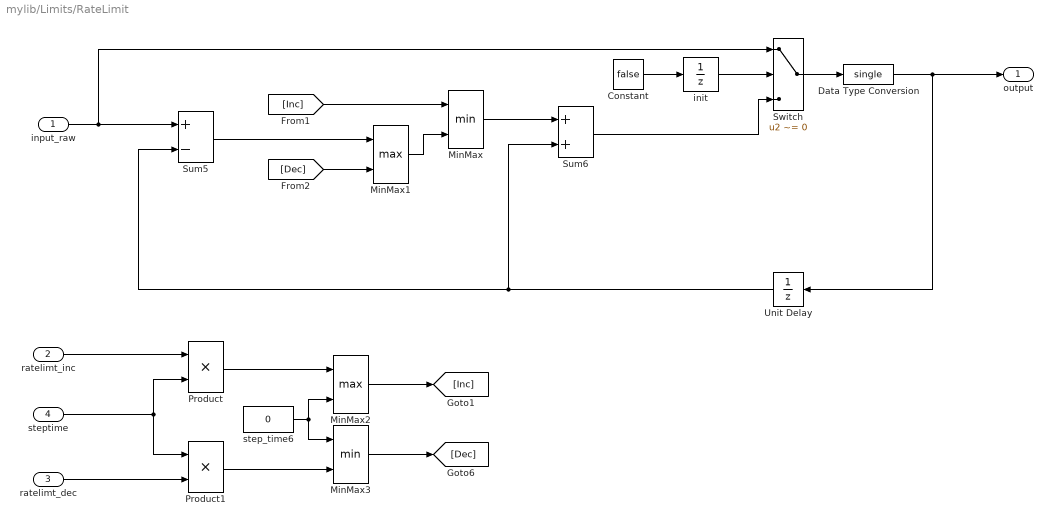
== system mylib/Limits/RateLimit ==
  input_raw : Inport  PortDimensions=1
  ratelimt_inc : Inport  Port=2  PortDimensions=1
  ratelimt_dec : Inport  Port=3  PortDimensions=1
  steptime : Inport  Port=4  PortDimensions=1
  Constant : Constant  Value=false
  Data Type Conversion : DataTypeConversion  OutDataTypeStr=single  RndMeth=Zero
  MinMax : MinMax  Inputs=2
  MinMax1 : MinMax  Function=max  Inputs=2
  MinMax2 : MinMax  Function=max  Inputs=2
  MinMax3 : MinMax  Inputs=2
  Product : Product  RndMeth=Zero
  Product1 : Product  RndMeth=Zero
  Sum5 : Sum  Inputs=+-
  Sum6 : Sum
  Switch : Switch  Criteria=u2 ~= 0
  Unit Delay : UnitDelay  InitialCondition=single(0)  SampleTime=-1
      settings: AttributesFormatString=<initial=%<x0>>\n<tsample=%<sampleTime>>
  init : UnitDelay  InitialCondition=true  SampleTime=-1
      settings: AttributesFormatString=<X0=%<X0>>
  step_time6 : Constant  Value=0  OutDataTypeStr=single
  output : Outport
  wires:
  ratelimt_dec/1 -> Product1/2
  steptime/1 -> Product1/1, Product/2
  Sum5/1 -> MinMax1/1
  [Dec] -> MinMax1/2
  [Inc] -> MinMax/1
  MinMax1/1 -> MinMax/2
  MinMax/1 -> Sum6/1
  input_raw/1 -> Sum5/1, Switch/1
  Unit Delay/1 -> Sum5/2, Sum6/2
  Product/1 -> MinMax2/1
  Product1/1 -> MinMax3/2
  step_time6/1 -> MinMax2/2, MinMax3/1
  MinMax2/1 -> [Inc]
  MinMax3/1 -> [Dec]
  ratelimt_inc/1 -> Product/1
  Constant/1 -> init/1
  Switch/1 -> Data Type Conversion/1
  init/1 -> Switch/2
  Sum6/1 -> Switch/3
  Data Type Conversion/1 -> Unit Delay/1, output/1

== system mylib/Memory/DoubleEdge_Detect ==
  flg_in : Inport
  Logical Operator : Logic  Operator=XOR  AllPortsSameDT=off  OutDataTypeStr=boolean
  Unit Delay : UnitDelay  SampleTime=-1
      settings: AttributesFormatString=<initial=%<x0>>\n<tsample=%<sampleTime>>
  flg_out : Outport
  wires:
  Unit Delay/1 -> Logical Operator/2
  flg_in/1 -> Logical Operator/1, Unit Delay/1
  Logical Operator/1 -> flg_out/1

== system mylib/Memory/Falling_Detect ==
  flg_in : Inport
  Logical Operator : Logic  AllPortsSameDT=off  OutDataTypeStr=boolean
  Logical Operator1 : Logic  Operator=NOT  AllPortsSameDT=off  OutDataTypeStr=boolean
  Unit Delay : UnitDelay  SampleTime=-1
      settings: AttributesFormatString=<initial=%<x0>>\n<tsample=%<sampleTime>>
  flg_out : Outport
  wires:
  Logical Operator/1 -> flg_out/1
  flg_in/1 -> Logical Operator1/1, Unit Delay/1
  Logical Operator1/1 -> Logical Operator/1
  Unit Delay/1 -> Logical Operator/2

== system mylib/Memory/Rising_Detect ==
  flg_in : Inport
  Logical Operator : Logic  AllPortsSameDT=off  OutDataTypeStr=boolean
  Logical Operator1 : Logic  Operator=NOT  AllPortsSameDT=off  OutDataTypeStr=boolean
  Unit Delay : UnitDelay  SampleTime=-1
      settings: AttributesFormatString=<initial=%<x0>>\n<tsample=%<sampleTime>>
  flg_out : Outport
  wires:
  Unit Delay/1 -> Logical Operator1/1
  flg_in/1 -> Unit Delay/1, Logical Operator/1
  Logical Operator/1 -> flg_out/1
  Logical Operator1/1 -> Logical Operator/2

== system mylib/Memory/SR_latch ==
  flg_set : Inport  OutDataTypeStr=boolean
      settings: AttributesFormatString=<tsample=%<sampletime>>
  flg_reset : Inport  Port=2  OutDataTypeStr=boolean
      settings: AttributesFormatString=<tsample=%<sampletime>>
  Logical Operator : Logic  Operator=OR  AllPortsSameDT=off  OutDataTypeStr=boolean
  Logical Operator1 : Logic  Operator=NOT  AllPortsSameDT=off  OutDataTypeStr=boolean
  Logical Operator3 : Logic  AllPortsSameDT=off  OutDataTypeStr=boolean
  Unit Delay : UnitDelay  InitialCondition=false  SampleTime=-1
      settings: AttributesFormatString=<initial=%<x0>>\n<tsample=%<sampletime>>
  flg_out : Outport  OutDataTypeStr=boolean
      settings: AttributesFormatString=<tsample=%<sampletime>>
  wires:
  Logical Operator3/1 -> flg_out/1, Unit Delay/1
  Unit Delay/1 -> Logical Operator/1
  Logical Operator1/1 -> Logical Operator3/2
  flg_reset/1 -> Logical Operator1/1
  flg_set/1 -> Logical Operator/2
  Logical Operator/1 -> Logical Operator3/1

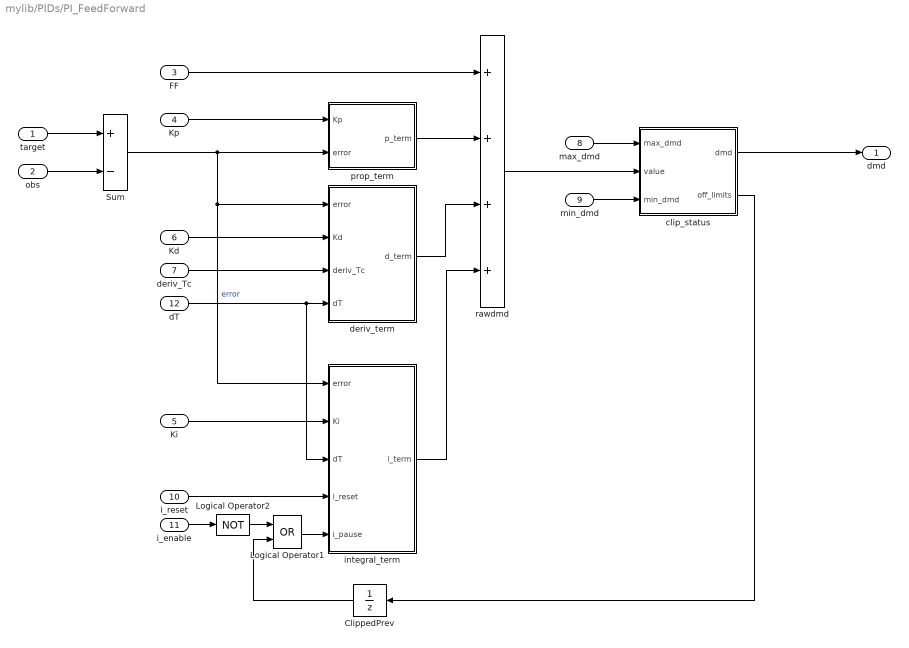
== system mylib/PIDs/PI_FeedForward ==
  target : Inport
  obs : Inport  Port=2
  FF : Inport  Port=3
  Kp : Inport  Port=4
  Ki : Inport  Port=5
  Kd : Inport  Port=6
  deriv_Tc : Inport  Port=7
  max_dmd : Inport  Port=8
  min_dmd : Inport  Port=9
  i_reset : Inport  Port=10
  i_enable : Inport  Port=11
  dT : Inport  Port=12
  ClippedPrev : UnitDelay  InitialCondition=false  SampleTime=-1
      settings: AttributesFormatString=<initial=%<x0>>\n<tsample=%<sampleTime>>
  Logical Operator1 : Logic  Operator=OR  AllPortsSameDT=off  OutDataTypeStr=boolean
  Logical Operator2 : Logic  Operator=NOT  AllPortsSameDT=off  OutDataTypeStr=boolean
  Sum : Sum  Inputs=+-  RndMeth=Zero
  clip_status : Subsystem
  deriv_term : Subsystem
  integral_term : Subsystem
  prop_term : Subsystem
  rawdmd : Sum  Inputs=++++  RndMeth=Zero
  dmd : Outport
  wires:
  FF/1 -> rawdmd/1
  target/1 -> Sum/1
  obs/1 -> Sum/2
  Kp/1 -> prop_term/1(Kp)
  Ki/1 -> integral_term/2(Ki)
  dT/1 -> integral_term/3(dT), deriv_term/4(dT)
  rawdmd/1 -> clip_status/2(value)
  prop_term/1(p_term) -> rawdmd/2
  integral_term/1(i_term) -> rawdmd/4
  max_dmd/1 -> clip_status/1(max_dmd)
  min_dmd/1 -> clip_status/3(min_dmd)
  clip_status/1(dmd) -> dmd/1
  clip_status/2(off_limits) -> ClippedPrev/1
  ClippedPrev/1 -> Logical Operator1/2
  i_reset/1 -> integral_term/4(i_reset)
  Sum/1 -> integral_term/1(error), deriv_term/1(error), prop_term/2(error)  "error"
  i_enable/1 -> Logical Operator2/1
  Logical Operator1/1 -> integral_term/5(i_pause)
  Logical Operator2/1 -> Logical Operator1/1
  deriv_term/1(d_term) -> rawdmd/3
  Kd/1 -> deriv_term/2(Kd)
  deriv_Tc/1 -> deriv_term/3(deriv_Tc)

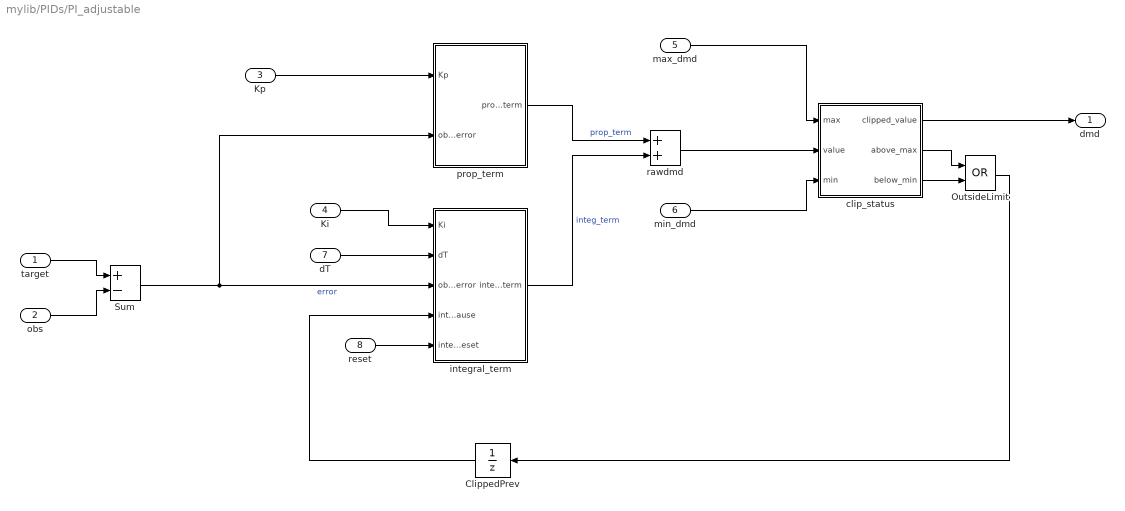
== system mylib/PIDs/PI_adjustable ==
  target : Inport
      settings: AttributesFormatString=<tsample=%<SampleTime>>
  obs : Inport  Port=2
      settings: AttributesFormatString=<tsample=%<SampleTime>>
  Kp : Inport  Port=3
      settings: AttributesFormatString=<tsample=%<SampleTime>>
  Ki : Inport  Port=4
      settings: AttributesFormatString=<tsample=%<SampleTime>>
  max_dmd : Inport  Port=5
      settings: AttributesFormatString=<tsample=%<SampleTime>>
  min_dmd : Inport  Port=6
      settings: AttributesFormatString=<tsample=%<SampleTime>>
  dT : Inport  Port=7
      settings: AttributesFormatString=<tsample=%<SampleTime>>
  reset : Inport  Port=8
      settings: AttributesFormatString=<tsample=%<SampleTime>>
  ClippedPrev : UnitDelay  InitialCondition=false  SampleTime=-1
      settings: AttributesFormatString=<initial=%<x0>>\n<tsample=%<sampleTime>>
  OutsideLimit : Logic  Operator=OR  AllPortsSameDT=off  OutDataTypeStr=boolean
  Sum : Sum  Inputs=+-  RndMeth=Zero
  clip_status : Subsystem
  integral_term : Subsystem
  prop_term : Subsystem
  rawdmd : Sum  RndMeth=Zero
  dmd : Outport
      settings: AttributesFormatString=<tsample=%<SampleTime>>
  wires:
  target/1 -> Sum/1
  obs/1 -> Sum/2
  Kp/1 -> prop_term/1(Kp)
  Ki/1 -> integral_term/1(Ki)
  dT/1 -> integral_term/2(dT)
  rawdmd/1 -> clip_status/2(value)
  prop_term/1(prop_term) -> rawdmd/1  "prop_term"
  integral_term/1(integ_term) -> rawdmd/2  "integ_term"
  max_dmd/1 -> clip_status/1(max)
  min_dmd/1 -> clip_status/3(min)
  clip_status/1(clipped_value) -> dmd/1
  clip_status/2(above_max) -> OutsideLimit/1
  clip_status/3(below_min) -> OutsideLimit/2
  OutsideLimit/1 -> ClippedPrev/1
  ClippedPrev/1 -> integral_term/4(integral_pause)
  reset/1 -> integral_term/5(integral_reset)
  Sum/1 -> prop_term/2(obs_error), integral_term/3(obs_error)  "error"

== system mylib/Switchs/Save_Value ==
  save_active : Inport
  u : Inport  Port=2
  RV : Inport  Port=3
  R : Inport  Port=4
  Logical Operator : Logic  Operator=NOT  AllPortsSameDT=off  OutDataTypeStr=boolean
  Selector : $bdroot/Switchs/Selector  SystemSampleTime=-1
  Unit Delay : UnitDelay  InitialCondition=initvalue  SampleTime=-1
      settings: AttributesFormatString=<initial=%<x0>>\n<tsample=%<sampleTime>>
  save_value : Outport
  wires:
  Selector/1 -> Unit Delay/1, save_value/1
  Unit Delay/1 -> Selector/5
  Logical Operator/1 -> Selector/1
  save_active/1 -> Logical Operator/1
  R/1 -> Selector/2
  RV/1 -> Selector/3
  u/1 -> Selector/4

== system mylib/Switchs/Selector ==
  E : Inport
  R : Inport  Port=2
  IV : Inport  Port=3
  u : Inport  Port=4
  z_last : Inport  Port=5
  Switch : Switch  Criteria=u2 ~= 0  Threshold=0.5  RndMeth=Zero
      settings: AttributesFormatString=<threshold=%<threshold>>\n<criteria=%<Criteria>>
  Switch1 : Switch  Criteria=u2 ~= 0  Threshold=0.5  RndMeth=Zero
      settings: AttributesFormatString=<threshold=%<threshold>>\n<criteria=%<Criteria>>
  y : Outport
  wires:
  Switch1/1 -> Switch/3
  R/1 -> Switch/2
  IV/1 -> Switch/1
  u/1 -> Switch1/1
  z_last/1 -> Switch1/3
  Switch/1 -> y/1
  E/1 -> Switch1/2

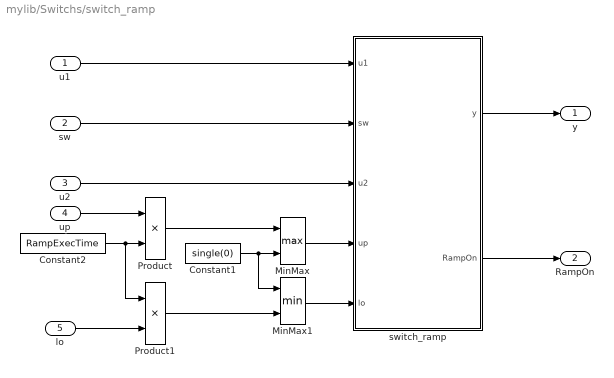
== system mylib/Switchs/switch_ramp ==
  u1 : Inport
  sw : Inport  Port=2
  u2 : Inport  Port=3
  up : Inport  Port=4
  lo : Inport  Port=5
  Constant1 : Constant  Value=single(0)  SampleTime=-1
      settings: AttributesFormatString=<tsample=%<SampleTime>>
  Constant2 : Constant  Value=RampExecTime  OutDataTypeStr=single  SampleTime=-1
  MinMax : MinMax  Function=max  Inputs=2  OutDataTypeStr=single  RndMeth=Zero
  MinMax1 : MinMax  Inputs=2  OutDataTypeStr=single  RndMeth=Zero
  Product : Product
  Product1 : Product
  switch_ramp : Subsystem
  y : Outport
  RampOn : Outport  Port=2
  wires:
  switch_ramp/2(RampOn) -> RampOn/1
  MinMax/1 -> switch_ramp/4(up)
  MinMax1/1 -> switch_ramp/5(lo)
  u2/1 -> switch_ramp/3(u2)
  sw/1 -> switch_ramp/2(sw)
  u1/1 -> switch_ramp/1(u1)
  switch_ramp/1(y) -> y/1
  up/1 -> Product/1
  lo/1 -> Product1/2
  Constant2/1 -> Product1/1, Product/2
  Product/1 -> MinMax/1
  Constant1/1 -> MinMax1/1, MinMax/2
  Product1/1 -> MinMax1/2

== system mylib/UintsConvert/G_to_mps2 ==
  u : Inport
  Constant : Constant  Value=G_2_MPS2  SampleTime=-1
      settings: AttributesFormatString=<tsample=%<SampleTime>>
  Product : Product  RndMeth=Zero
  y : Outport
  wires:
  Constant/1 -> Product/2
  u/1 -> Product/1  "u"
  Product/1 -> y/1  "y"

== system mylib/UintsConvert/bar2pa ==
  u : Inport
  Constant : Constant  Value=BAR_2_Pa  SampleTime=-1
      settings: AttributesFormatString=<tsample=%<SampleTime>>
  Product : Product  RndMeth=Zero
  y : Outport
  wires:
  Product/1 -> y/1  "y"
  Constant/1 -> Product/2
  u/1 -> Product/1  "u"

== system mylib/UintsConvert/cc_2_m3 ==
  u : Inport
  Constant : Constant  Value=CC_2_M3  SampleTime=-1
      settings: AttributesFormatString=<tsample=%<SampleTime>>
  Product : Product  RndMeth=Zero
  y : Outport
  wires:
  u/1 -> Product/1  "u"
  Constant/1 -> Product/2
  Product/1 -> y/1  "y"

== system mylib/UintsConvert/ccprev_2_m3prad ==
  u : Inport
  Constant : Constant  Value=CCpREV_2_M3pRAD  SampleTime=-1
      settings: AttributesFormatString=<tsample=%<SampleTime>>
  Product : Product  RndMeth=Zero
  y : Outport
  wires:
  u/1 -> Product/1  "u"
  Constant/1 -> Product/2
  Product/1 -> y/1  "y"

== system mylib/UintsConvert/deg2rad ==
  u : Inport
  Constant : Constant  Value=DEG_2_RAD  SampleTime=-1
      settings: AttributesFormatString=<tsample=%<SampleTime>>
  Product : Product  RndMeth=Zero
  y : Outport
  wires:
  Constant/1 -> Product/2
  Product/1 -> y/1  "y"
  u/1 -> Product/1  "u"

== system mylib/UintsConvert/knots2kph ==
  u : Inport
  Constant : Constant  Value=KNOTS_2_KPH  SampleTime=-1
      settings: AttributesFormatString=<tsample=%<SampleTime>>
  Product : Product  RndMeth=Zero
  y : Outport
  wires:
  u/1 -> Product/1  "u"
  Product/1 -> y/1  "y"
  Constant/1 -> Product/2

== system mylib/UintsConvert/kph2knots ==
  u : Inport
  Constant : Constant  Value=KPH_2_KNOTS  SampleTime=-1
      settings: AttributesFormatString=<tsample=%<SampleTime>>
  Product : Product  RndMeth=Zero
  y : Outport
  wires:
  Product/1 -> y/1  "y"
  u/1 -> Product/1  "u"
  Constant/1 -> Product/2

== system mylib/UintsConvert/kph2mps ==
  u : Inport
  Constant : Constant  Value=KPH_2_MPS  SampleTime=-1
      settings: AttributesFormatString=<tsample=%<SampleTime>>
  Product : Product  RndMeth=Zero
  y : Outport
  wires:
  Product/1 -> y/1  "y"
  u/1 -> Product/1  "u"
  Constant/1 -> Product/2

== system mylib/UintsConvert/kxx2xx ==
  u : Inport
  Constant : Constant  Value=kXX_2_XX  SampleTime=-1
      settings: AttributesFormatString=<tsample=%<SampleTime>>
  Product : Product  RndMeth=Zero
  y : Outport
  wires:
  u/1 -> Product/1  "u"
  Product/1 -> y/1  "y"
  Constant/1 -> Product/2

== system mylib/UintsConvert/m3_2_cc ==
  u : Inport
  Constant : Constant  Value=M3_2_CC  SampleTime=-1
      settings: AttributesFormatString=<tsample=%<SampleTime>>
  Product : Product  RndMeth=Zero
  y : Outport
  wires:
  Product/1 -> y/1  "y"
  Constant/1 -> Product/2
  u/1 -> Product/1  "u"

== system mylib/UintsConvert/m3prad_2_ccprev ==
  u : Inport
  Constant : Constant  Value=M3pRAD_2_CCpREV  SampleTime=-1
      settings: AttributesFormatString=<tsample=%<SampleTime>>
  Product : Product  RndMeth=Zero
  y : Outport
  wires:
  Product/1 -> y/1  "y"
  Constant/1 -> Product/2
  u/1 -> Product/1  "u"

== system mylib/UintsConvert/mps2_to_G ==
  u : Inport
  Constant : Constant  Value=MPS2_2_G  SampleTime=-1
      settings: AttributesFormatString=<tsample=%<SampleTime>>
  Product : Product  RndMeth=Zero
  y : Outport
  wires:
  Product/1 -> y/1  "y"
  u/1 -> Product/1  "u"
  Constant/1 -> Product/2

== system mylib/UintsConvert/mps2kph ==
  u : Inport
  Constant : Constant  Value=MPS_2_KPH  SampleTime=-1
      settings: AttributesFormatString=<tsample=%<SampleTime>>
  Product : Product  RndMeth=Zero
  y : Outport
  wires:
  u/1 -> Product/1  "u"
  Product/1 -> y/1  "y"
  Constant/1 -> Product/2

== system mylib/UintsConvert/pa2bar ==
  u : Inport
  Constant : Constant  Value=Pa_2_BAR  SampleTime=-1
      settings: AttributesFormatString=<tsample=%<SampleTime>>
  Product : Product  RndMeth=Zero
  y : Outport
  wires:
  u/1 -> Product/1  "u"
  Constant/1 -> Product/2
  Product/1 -> y/1  "y"

== system mylib/UintsConvert/rad2deg ==
  u : Inport
  Constant : Constant  Value=RAD_2_DEG  SampleTime=-1
      settings: AttributesFormatString=<tsample=%<SampleTime>>
  Product : Product  RndMeth=Zero
  y : Outport
  wires:
  Constant/1 -> Product/2
  u/1 -> Product/1  "u"
  Product/1 -> y/1  "y"

== system mylib/UintsConvert/radps2rpm ==
  u : Inport
  Constant : Constant  Value=RADpS_2_RPM  SampleTime=-1
      settings: AttributesFormatString=<tsample=%<SampleTime>>
  Product : Product  OutDataTypeStr=single  RndMeth=Zero
  y : Outport
  wires:
  u/1 -> Product/1  "u"
  Product/1 -> y/1  "y"
  Constant/1 -> Product/2

== system mylib/UintsConvert/rpm2radps ==
  u : Inport
  Constant : Constant  Value=RPM_2_RADpS  SampleTime=-1
      settings: AttributesFormatString=<tsample=%<SampleTime>>
  Product : Product  RndMeth=Zero
  y : Outport
  wires:
  Product/1 -> y/1  "y"
  u/1 -> Product/1  "u"
  Constant/1 -> Product/2

== system mylib/UintsConvert/xx2kxx ==
  u : Inport
  Constant : Constant  Value=XX_2_kXX  SampleTime=-1
      settings: AttributesFormatString=<tsample=%<SampleTime>>
  Product : Product  RndMeth=Zero
  y : Outport
  wires:
  u/1 -> Product/1  "u"
  Constant/1 -> Product/2
  Product/1 -> y/1  "y"

== system mylib/Universals/Atomic Subsystem ==
  In1 : Inport
      settings: AttributesFormatString=<tsample=%<SampleTime>>
  Out1 : Outport
      settings: AttributesFormatString=<tsample=%<SampleTime>>
  wires:
  In1/1 -> Out1/1

== system mylib/Universals/CodeReuseSubsystem ==
  In1 : Inport
      settings: AttributesFormatString=<tsample=%<SampleTime>>
  Out1 : Outport
      settings: AttributesFormatString=<tsample=%<SampleTime>>
  wires:
  In1/1 -> Out1/1

== system mylib/Universals/Compare To Constant ==
  u : Inport
      settings: AttributesFormatString=<tsample=%<SampleTime>>
  Compare : RelationalOperator  Operator===  OutDataTypeStr=boolean  ZeroCross=off  RndMeth=Nearest  InputSameDT=on
  Constant : Constant  DisableCoverage=on  Value=const  OutDataTypeStr=Inherit: Inherit via back propagation  SampleTime=-1
      settings: AttributesFormatString=<tsample=%<SampleTime>>
  y : Outport
      settings: AttributesFormatString=<tsample=%<SampleTime>>
  wires:
  Compare/1 -> y/1  "y"
  Constant/1 -> Compare/2
  u/1 -> Compare/1  "u"

== system mylib/Universals/DocBlockDescription ==
  EmptySubsystem : Subsystem

== system mylib/Universals/DocBlockHistory ==
  EmptySubsystem : Subsystem

== system mylib/Universals/Function-Call Subsystem ==
  In1 : Inport
      settings: AttributesFormatString=<tsample=%<SampleTime>>
  function : TriggerPort  TriggerType=function-call  VariantControl=(inherit)
  Out1 : Outport
      settings: AttributesFormatString=<tsample=%<SampleTime>>
  wires:
  In1/1 -> Out1/1

== system mylib/Universals/If Action Subsystem ==
  In1 : Inport
      settings: AttributesFormatString=<tsample=%<SampleTime>>
  Action Port : ActionPort  ActionType=then
  Out1 : Outport
      settings: AttributesFormatString=<tsample=%<SampleTime>>
  wires:
  In1/1 -> Out1/1

== system mylib/Universals/ReqId ==
